simulink model "sine_hydraulic_fmu"  (R2024b)
settings: Solver=VariableStepAuto  StartTime=0.0  StopTime=100  RelTol=1e-6
settings Model: Creator=thogan1  LastModifiedBy=thogan1

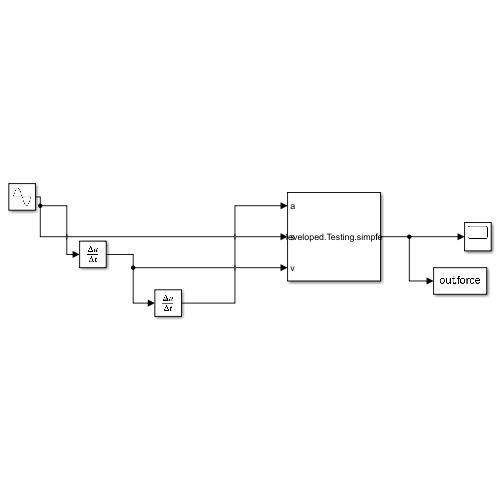
[thumbnail: Simulink's stored preview of the top-level diagram]
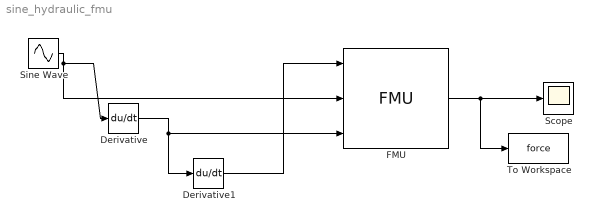
== system sine_hydraulic_fmu ==
  Derivative : Derivative
  Derivative1 : Derivative
  FMU : FMU  FMUName=simple_FMU_force_fmu.fmu  FMUMode=ModelExchange  FMUInitializeEnumObject=off  doubleActingCylinder=struct('CHeadExLeakage',0.0,'CInLeakage',0.0,'CRodExLeakage',0.0,'Cst',0.5,'Cv',1.0,'a_init',0.0,'boreDiameter',0.04,'closedLength',1e-4,'cylinderChamberHead',struct('residualVolume',3e-4,'accumulatorEnable',boolean(false)),'cylinderChamberRod',struct('residualVolume',3e-4,'accumulatorEnable',boolean(false)),'damper',struct('s_nominal',1e-4),'damping',1e4,'dp_nom',1e4,'endOfTravelDistance',0.01,'f_c',5.0,'f_st',10.0,'maxPressure',2e8,'p_init',1e6,'piston',struct('L',0.0),'pistonRodMass',1.0,'q_nom',0.01,'rodDiameter',0.029,'s_init',0.0,'stopDamping',1e12,'stopStiffness',1e9,'strokeLength',3.0,'v_init',0.0)  environment=struct('T_ambient',288.15,'p_ambient',101325.0)  fixed=struct('s0',0.0)  laminarRestriction=struct('L',10.0,'Re_laminar',2000.0)  laminarRestriction1=struct('L',10.0,'Re_laminar',2000.0)  system=struct('T_ambient',293.15,'dp_small',1.0,'eps_m_flow',1e-4,'m_flow_small',0.01,'m_flow_start',0.0,'p_ambient',101325.0)  mask(OpenHydraulics.Developed.Testing.simple_FMU_force_fmu [Model Exchange, v2.0]){}
      settings: MultithreadedSim=off
      mask Display:
      | disp('OpenHydraulics.Developed.Testing.simple_FMU_force_fmu');
      | port_label('output',1,'f');
      | port_label('input',1,'a');
      | port_label('input',2,'s');
      | port_label('input',3,'v');
  Scope : Scope
  Sine Wave : Sin  Bias=1.5  Frequency=2*pi/17.7  SampleTime=0
  To Workspace : ToWorkspace  VariableName=force  SaveFormat=Timeseries  SampleTime=-1
  wires:
  Sine Wave/1 -> FMU/2, Derivative/1
  Derivative/1 -> FMU/3, Derivative1/1
  FMU/1 -> To Workspace/1, Scope/1
  Derivative1/1 -> FMU/1
